simulink model "SimplePendulumWithoutFeedback"  (R2017b)
settings: Solver=ode45  StartTime=0.0  StopTime=T  RelTol=1e-3  EnableMultiTasking=on
undefined symbols (not defined in the file or in its folder): b, g, Jr, m, r, tauBar, theta0
settings Model: Creator=mauricio  LastModifiedBy=mauricio
settings DataIOCC: LimitDataPoints=on  SaveFormat=Array  SignalLoggingSaveFormat=ModelDataLogs
settings OptimizationCC: ExpressionDepthLimit=2147483647  LifeSpan=inf
settings DebuggingCC: UnderspecifiedInitializationDetection=Classic  MergeDetectMultiDrivingBlocksExec=none  FcnCallInpInsideContextMsg=warning  StateNameClashWarn=warning  SFUnexpectedBacktrackingDiag=warning  SFNoUnconditionalDefaultTransitionDiag=warning  SFExecutionAtInitializationDiag=none
settings HardwareCC: ProdBitPerPointer=32  ProdBitPerSizeT=32  ProdBitPerPtrDiffT=32  ProdLargestAtomicFloat=None  ProdIntDivRoundTo=Undefined  ProdEndianess=Unspecified  ProdWordSize=32  ProdHWDeviceType=32-bit Generic
settings ModelReferenceCC: PropagateSignalLabelsOutOfModel=off
settings CodeAppCC: StateflowObjectComments=on
settings GRTTargetCC: TargetLangStandard=C89/C90 (ANSI)  GeneratePreprocessorConditionals=Disable all  CombineOutputUpdateFcns=off  GRTInterface=on
settings ConfigComp: CovMetricSettings=dw  CovHtmlReporting=on  CovSaveCumulativeToWorkspaceVar=on  CovSaveSingleToWorkspaceVar=on  CovExternalEMLEnable=off  CovSFcnEnable=off

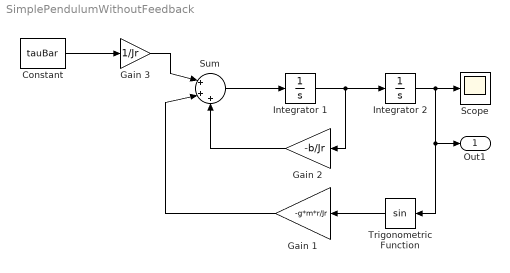
== system SimplePendulumWithoutFeedback ==
  Constant : Constant  Value=tauBar
  Gain 1 : Gain  Gain=-g*m*r/Jr
  Gain 2 : Gain  Gain=-b/Jr
  Gain 3 : Gain  Gain=1/Jr
  Integrator 1 : Integrator
  Integrator 2 : Integrator  InitialCondition=theta0
  Scope : Scope
  Sum : Sum  Inputs=|+++
  Trigonometric Function : Trigonometry
  Out1 : Outport
  wires:
  Integrator 1/1 -> Integrator 2/1, Gain 2/1
  Integrator 2/1 -> Scope/1, Trigonometric Function/1, Out1/1
  Trigonometric Function/1 -> Gain 1/1
  Sum/1 -> Integrator 1/1
  Gain 2/1 -> Sum/3
  Gain 1/1 -> Sum/2
  Gain 3/1 -> Sum/1
  Constant/1 -> Gain 3/1
